simulink model "Controller_Pioneer3DXAssembly_org"  (Simulink 10.0)
settings: Solver=ode45  StartTime=0.0  StopTime=200  RelTol=1e-3  EnableMultiTasking=on
InitFcn:
  | load WorldLUTData.mat
  | r = 0.095; %Wheel radius
  | b = 0.33; %Wheel base
undefined symbols (not defined in the file): World_LUT, X, Y, Z
libraries: sm_lib x35, nesl_utility x19, fl_lib x3, fl_ps_legacy_lib x3, vrlib x2
(part 1 of 2)
settings Model: Creator=sseshadr  LastModifiedBy=bhisma
settings DataIOCC: LimitDataPoints=on
settings DebuggingCC: SolverPrmCheckMsg=warning
settings GRTTargetCC: GeneratePreprocessorConditionals=Disable all  CombineOutputUpdateFcns=on  GRTInterface=off
settings ConfigComp: CovExternalEMLEnable=off
settings SimscapeCC: SimscapeNormalizeSystem=off
settings ConfigurationSet: Description=SimMechanics 2G
settings ExplorerConfigSet: SimMechanicsOpenEditorOnUpdate=off

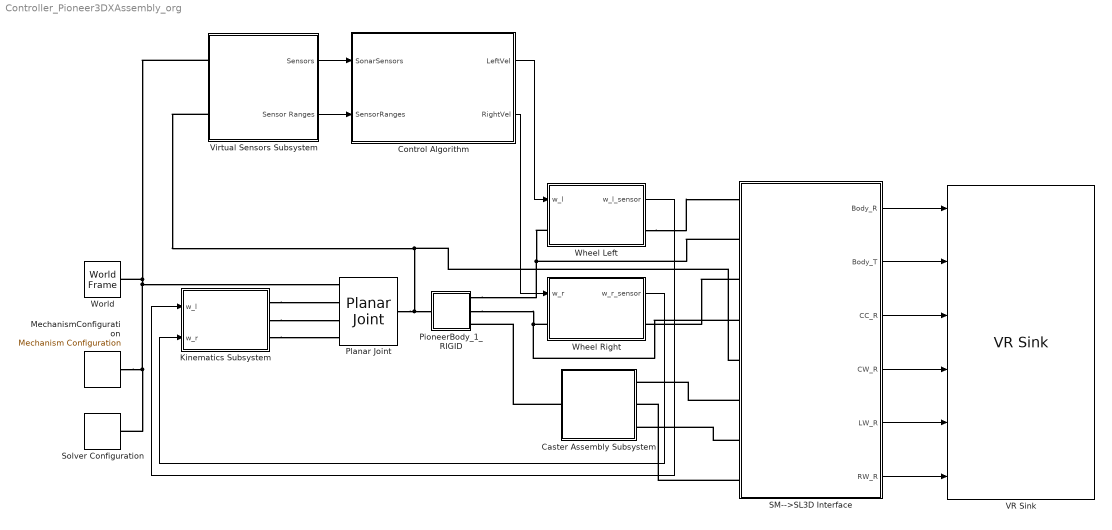
== system Controller_Pioneer3DXAssembly_org ==
  Caster Assembly Subsystem : Subsystem
  Control Algorithm : Stateflow chart  TreatAsAtomicUnit=on  mask{v0=1}
      mask prompts: v0 "Wheel Angular Velocity"
  Kinematics Subsystem : Subsystem
  MechanismConfiguration : sm_lib/Utilities/Mechanism Configuration  UniformGravity=Constant  GravityVector=[0 0 -9.81]  GravityUnits=m/s^2  LinearizationDelta=0.001
  PioneerBody_1_RIGID : Subsystem
  Planar Joint : sm_lib/Joints/Planar Joint  JointMode=Normal  SenseConstraintForce=off  SenseConstraintForceX=off  SenseConstraintForceY=off  SenseConstraintForceZ=off  SenseConstraintTorque=off  SenseConstraintTorqueX=off  SenseConstraintTorqueY=off  SenseConstraintTorqueZ=off  SenseTotalForce=off  SenseTotalForceX=off  SenseTotalForceY=off  SenseTotalForceZ=off  SenseTotalTorque=off  SenseTotalTorqueX=off  SenseTotalTorqueY=off  SenseTotalTorqueZ=off  CompositeWrenchDir=FollowerOnBase  CompositeWrenchFrame=BaseFrame  PxEquilibriumPosition=0  PxEquilibriumPositionUnits=m  PxSpringStiffness=0  PxSpringStiffnessUnits=N/m  PxDampingCoefficient=0  PxDampingCoefficientUnits=N/(m/s)  PxTorqueActuationMode=ComputedTorque  PxMotionActuationMode=InputMotion  PxSensePosition=off  PxSenseVelocity=off  PxSenseAcceleration=off  PxSenseTorqueForce=off  PxSenseLowerLimitTorqueForce=off  PxSenseUpperLimitTorqueForce=off  PxLowerLimitSpecify=off  PxLowerLimitBound=-1  PxLowerLimitBoundUnits=m  PxLowerLimitStiffness=1e6  PxLowerLimitStiffnessUnits=N/m  PxLowerLimitDamping=1e3  PxLowerLimitDampingUnits=N/(m/s)  PxLowerLimitTransitionRegionWidth=1e-4  PxLowerLimitTransitionRegionWidthUnits=m  PxUpperLimitSpecify=off  PxUpperLimitBound=1  PxUpperLimitBoundUnits=m  PxUpperLimitStiffness=1e6  PxUpperLimitStiffnessUnits=N/m  PxUpperLimitDamping=1e3  PxUpperLimitDampingUnits=N/(m/s)  PxUpperLimitTransitionRegionWidth=1e-4  PxUpperLimitTransitionRegionWidthUnits=m  PxPositionTargetSpecify=off  PxPositionTargetPriority=High  PxPositionTargetValue=0  PxPositionTargetValueUnits=m  PxVelocityTargetSpecify=off  PxVelocityTargetPriority=High  PxVelocityTargetValue=0  PxVelocityTargetValueUnits=m/s  PyEquilibriumPosition=0  PyEquilibriumPositionUnits=m  PySpringStiffness=0  PySpringStiffnessUnits=N/m  PyDampingCoefficient=0  PyDampingCoefficientUnits=N/(m/s)  PyTorqueActuationMode=ComputedTorque  PyMotionActuationMode=InputMotion  PySensePosition=off  PySenseVelocity=off  PySenseAcceleration=off  PySenseTorqueForce=off  PySenseLowerLimitTorqueForce=off  PySenseUpperLimitTorqueForce=off  PyLowerLimitSpecify=off  PyLowerLimitBound=-1  PyLowerLimitBoundUnits=m  PyLowerLimitStiffness=1e6  PyLowerLimitStiffnessUnits=N/m  PyLowerLimitDamping=1e3  PyLowerLimitDampingUnits=N/(m/s)  PyLowerLimitTransitionRegionWidth=1e-4  PyLowerLimitTransitionRegionWidthUnits=m  PyUpperLimitSpecify=off  PyUpperLimitBound=1  PyUpperLimitBoundUnits=m  PyUpperLimitStiffness=1e6  PyUpperLimitStiffnessUnits=N/m  PyUpperLimitDamping=1e3  PyUpperLimitDampingUnits=N/(m/s)  PyUpperLimitTransitionRegionWidth=1e-4  PyUpperLimitTransitionRegionWidthUnits=m  PyPositionTargetSpecify=off  PyPositionTargetPriority=High  PyPositionTargetValue=0  PyPositionTargetValueUnits=m  PyVelocityTargetSpecify=off  PyVelocityTargetPriority=High  PyVelocityTargetValue=0  PyVelocityTargetValueUnits=m/s  RzEquilibriumPosition=0  RzEquilibriumPositionUnits=deg  RzSpringStiffness=0  RzSpringStiffnessUnits=N*m/deg  RzDampingCoefficient=0  RzDampingCoefficientUnits=N*m/(deg/s)  RzTorqueActuationMode=ComputedTorque  RzMotionActuationMode=InputMotion  RzSensePosition=off  RzSenseVelocity=off  RzSenseAcceleration=off  RzSenseTorqueForce=off  RzSenseLowerLimitTorqueForce=off  RzSenseUpperLimitTorqueForce=off  RzLowerLimitSpecify=off  RzLowerLimitBound=-90  RzLowerLimitBoundUnits=deg  RzLowerLimitStiffness=1e4  RzLowerLimitStiffnessUnits=N*m/deg  RzLowerLimitDamping=10  RzLowerLimitDampingUnits=N*m/(deg/s)  RzLowerLimitTransitionRegionWidth=0.1  RzLowerLimitTransitionRegionWidthUnits=deg  RzUpperLimitSpecify=off  RzUpperLimitBound=90  RzUpperLimitBoundUnits=deg  RzUpperLimitStiffness=1e4  RzUpperLimitStiffnessUnits=N*m/deg  RzUpperLimitDamping=10  RzUpperLimitDampingUnits=N*m/(deg/s)  RzUpperLimitTransitionRegionWidth=0.1  RzUpperLimitTransitionRegionWidthUnits=deg  RzPositionTargetSpecify=off  RzPositionTargetPriority=High  RzPositionTargetValue=0  RzPositionTargetValueUnits=deg  RzVelocityTargetSpecify=off  RzVelocityTargetPriority=High  RzVelocityTargetValue=0  RzVelocityTargetValueUnits=deg/s
  SM-->SL3D Interface : Subsystem
  Solver Configuration : nesl_utility/Solver Configuration  PhysicalDomain=network_engine_domain  SubClassName=solver  LeftPortType=input  RightPortType=generic  Tones=[]  Harmonics=[]  SimulateNoise=off  Profile=off  UseLocalSampling=off  EnableSwitchedLinearOptims=on  FrequencyDomain=off  UseCCode=off  RelTol=0.001  AbsTol=1e-06  MinStep=1e-09  ToWorkspace=off  RevertToSquareIcSolve=off  NumHomotopyIterations=100  PhasorMode=off  PhasorModeNumHarmonics=1  DoDC=off  ResidualTolerance=1e-09  UseLocalSolver=off  LocalSolverChoice=NE_BACKWARD_EULER_ADVANCER  LocalSolverSampleTime=0.001  DoFixedCost=off  MaxNonlinIter=3  MaxModeIter=2  LinearAlgebra=Sparse  EquationFormulation=NE_TIME_EF  DelaysMemoryBudget=1024  AutomaticFiltering=on  FilteringTimeConstant=0.001  PartitionStorageMethod=AS_NEEDED  PartitionMemoryBudget=1024  PartitionMethod=FAST
  VR Sink : vrlib/VR Sink  InstantiateOnLoad=on  SampleTime=0.1  ViewEnable=on  RemoteChange=off  RemoteView=off  FieldsWritten=Body.rotation.4.1.1.double#Body.translation.3.1.1.double#CasterClamp.rotation.4.1.1.double#CasterWheel.rotation.4.1.1.double#LeftWheel.rotation.4.1.1.double#RightWheel.rotation.4.1.1.double  WorldFileName=PioneerWorldColor.wrl  AutoView=off  VideoDimensions=[]  AllowVariableSize=off  FigureProperties="{'Position', 'Name', 'Viewpoint', 'CameraBound', 'CameraDirection', 'CameraPosition', 'CameraUpVector', 'ZoomFactor', 'Antialiasing', 'Headlight', 'Lighting', 'NavPanel', 'StatusBar', 'ToolBar', 'Textures', 'Transparency', 'Triad', 'Wireframe', 'NavZones', 'NavMode', 'NavSpeed', 'CaptureFileFormat', 'CaptureFileName', 'Record2DCompressMethod', 'Record2DCompressQuality', 'Record2D', 'Record2DFileName', 'Record2DFPS'; [9.6500000000000000e+02   7.0000000000000000e+01   9.5200000000000000e+02   1.0310000000000000e+03], '', 'Env Front Near', 'on', [0.0000000000000000e+00   0.0000000000000000e+00  -1.0000000000000000e+00], [0.0000000000000000e+00   0.0000000000000000e+00   0.0000000000000000e+00], [0.0000000000000000e+00   1.0000000000000000e+00   0.0000000000000000e+00], [1.0000000000000000e+00], 'on', 'on', 'on', 'halfbar', 'on', 'on', 'on', 'on', 'none', 'off', 'off', 'fly', 'normal', 'tif', '%f_anim_%n.tif', 'auto', [7.5000000000000000e+01], 'off', '%f_anim_%n.avi', [1.5000000000000000e+01]}"
      settings: SourceProductName=Simulink
  Virtual Sensors Subsystem : Subsystem  mask{r_range=[450;500;500;500;500;500;500;450]}
      mask prompts: r_range "Range"
      mask DialogControl DescGroupVar Prompt: Virtual Sensors Subsystem
      mask DialogControl DescTextVar Prompt: Enter SONAR Range for the front sensors left to right as an array for in millimeters for e.g. [250;500;500;500;500;500;500;250]
  Wheel Left : Subsystem
  Wheel Right : Subsystem
  World : sm_lib/Frames and Transforms/World Frame
  wires:
  Control Algorithm/1(LeftVel) -> Wheel Left/1(w_l)
  Control Algorithm/2(RightVel) -> Wheel Right/1(w_r)
  Wheel Left/1(w_l_sensor) -> Kinematics Subsystem/1(w_l)
  Wheel Right/1(w_r_sensor) -> Kinematics Subsystem/2(w_r)
  Virtual Sensors Subsystem/1(Sensors) -> Control Algorithm/1(SonarSensors)
  Virtual Sensors Subsystem/2(Sensor Ranges) -> Control Algorithm/2(SensorRanges)
  SM-->SL3D Interface/1(Body_R) -> VR Sink/1
  SM-->SL3D Interface/6(RW_R) -> VR Sink/6
  SM-->SL3D Interface/5(LW_R) -> VR Sink/5
  SM-->SL3D Interface/3(CC_R) -> VR Sink/3
  SM-->SL3D Interface/4(CW_R) -> VR Sink/4
  SM-->SL3D Interface/2(Body_T) -> VR Sink/2
  connections:
  MechanismConfiguration/RConn1 -- Virtual Sensors Subsystem/LConn1 -- World/RConn1 -- Planar Joint/LConn1 -- Solver Configuration/RConn1
  PioneerBody_1_RIGID/RConn2 -- SM-->SL3D Interface/LConn4 -- Wheel Right/LConn1
  PioneerBody_1_RIGID/RConn1 -- Wheel Left/LConn1 -- SM-->SL3D Interface/LConn2
  Planar Joint/RConn1 -- SM-->SL3D Interface/LConn5 -- Virtual Sensors Subsystem/LConn2 -- PioneerBody_1_RIGID/LConn1
  Caster Assembly Subsystem/LConn1 -- PioneerBody_1_RIGID/RConn3
  Kinematics Subsystem/RConn1 -- Planar Joint/LConn2
  Kinematics Subsystem/RConn2 -- Planar Joint/LConn3
  Kinematics Subsystem/RConn3 -- Planar Joint/LConn4
  Wheel Left/RConn1 -- SM-->SL3D Interface/LConn1
  SM-->SL3D Interface/LConn3 -- Wheel Right/RConn1
  SM-->SL3D Interface/LConn6 -- Caster Assembly Subsystem/RConn1
  SM-->SL3D Interface/LConn8 -- Caster Assembly Subsystem/RConn2
  SM-->SL3D Interface/LConn7 -- Caster Assembly Subsystem/RConn3

== system Controller_Pioneer3DXAssembly_org/Caster Assembly Subsystem ==
  CasterWheelBody_1_RIGID : Subsystem
  CasterWheelClamp_1_RIGID : Subsystem
  Revolute : sm_lib/Joints/Revolute Joint  JointMode=Normal  SenseConstraintForce=off  SenseConstraintForceX=off  SenseConstraintForceY=off  SenseConstraintForceZ=off  SenseConstraintTorque=off  SenseConstraintTorqueX=off  SenseConstraintTorqueY=off  SenseConstraintTorqueZ=off  SenseTotalForce=off  SenseTotalForceX=off  SenseTotalForceY=off  SenseTotalForceZ=off  SenseTotalTorque=off  SenseTotalTorqueX=off  SenseTotalTorqueY=off  SenseTotalTorqueZ=off  CompositeWrenchDir=FollowerOnBase  CompositeWrenchFrame=BaseFrame  EquilibriumPosition=0  EquilibriumPositionUnits=rad  SpringStiffness=0  SpringStiffnessUnits=m*N/rad  DampingCoefficient=0  DampingCoefficientUnits=m*s*N/rad  TorqueActuationMode=NoTorque  MotionActuationMode=ComputedMotion  SensePosition=off  SenseVelocity=off  SenseAcceleration=off  SenseTorqueForce=off  SenseLowerLimitTorqueForce=off  SenseUpperLimitTorqueForce=off  LowerLimitSpecify=off  LowerLimitBound=-90  LowerLimitBoundUnits=deg  LowerLimitStiffness=1e4  LowerLimitStiffnessUnits=N*m/deg  LowerLimitDamping=10  LowerLimitDampingUnits=N*m/(deg/s)  LowerLimitTransitionRegionWidth=0.1  LowerLimitTransitionRegionWidthUnits=deg  UpperLimitSpecify=off  UpperLimitBound=90  UpperLimitBoundUnits=deg  UpperLimitStiffness=1e4  UpperLimitStiffnessUnits=N*m/deg  UpperLimitDamping=10  UpperLimitDampingUnits=N*m/(deg/s)  UpperLimitTransitionRegionWidth=0.1  UpperLimitTransitionRegionWidthUnits=deg  PositionTargetSpecify=on  PositionTargetPriority=Low  PositionTargetValue=0.2241061767810246  PositionTargetValueUnits=deg  VelocityTargetSpecify=off  VelocityTargetPriority=High  VelocityTargetValue=0  VelocityTargetValueUnits=deg/s
  Revolute1 : sm_lib/Joints/Revolute Joint  JointMode=Normal  SenseConstraintForce=off  SenseConstraintForceX=off  SenseConstraintForceY=off  SenseConstraintForceZ=off  SenseConstraintTorque=off  SenseConstraintTorqueX=off  SenseConstraintTorqueY=off  SenseConstraintTorqueZ=off  SenseTotalForce=off  SenseTotalForceX=off  SenseTotalForceY=off  SenseTotalForceZ=off  SenseTotalTorque=off  SenseTotalTorqueX=off  SenseTotalTorqueY=off  SenseTotalTorqueZ=off  CompositeWrenchDir=FollowerOnBase  CompositeWrenchFrame=BaseFrame  EquilibriumPosition=0  EquilibriumPositionUnits=rad  SpringStiffness=0  SpringStiffnessUnits=m*N/rad  DampingCoefficient=0  DampingCoefficientUnits=m*s*N/rad  TorqueActuationMode=NoTorque  MotionActuationMode=ComputedMotion  SensePosition=off  SenseVelocity=off  SenseAcceleration=off  SenseTorqueForce=off  SenseLowerLimitTorqueForce=off  SenseUpperLimitTorqueForce=off  LowerLimitSpecify=off  LowerLimitBound=-90  LowerLimitBoundUnits=deg  LowerLimitStiffness=1e4  LowerLimitStiffnessUnits=N*m/deg  LowerLimitDamping=10  LowerLimitDampingUnits=N*m/(deg/s)  LowerLimitTransitionRegionWidth=0.1  LowerLimitTransitionRegionWidthUnits=deg  UpperLimitSpecify=off  UpperLimitBound=90  UpperLimitBoundUnits=deg  UpperLimitStiffness=1e4  UpperLimitStiffnessUnits=N*m/deg  UpperLimitDamping=10  UpperLimitDampingUnits=N*m/(deg/s)  UpperLimitTransitionRegionWidth=0.1  UpperLimitTransitionRegionWidthUnits=deg  PositionTargetSpecify=on  PositionTargetPriority=Low  PositionTargetValue=0.06600758954149441  PositionTargetValueUnits=deg  VelocityTargetSpecify=off  VelocityTargetPriority=High  VelocityTargetValue=0  VelocityTargetValueUnits=deg/s
  CWCA : PMIOPort  Side=Left
  CWC : PMIOPort  Port=2  Side=Right
  CWBA : PMIOPort  Port=3  Side=Right
  CWB : PMIOPort  Port=4  Side=Right
  connections:
  Revolute1/LConn1 -- CWBA/RConn1 -- CasterWheelClamp_1_RIGID/RConn1
  CWCA/RConn1 -- Revolute/LConn1
  Revolute1/RConn1 -- CWB/RConn1 -- CasterWheelBody_1_RIGID/LConn1
  Revolute/RConn1 -- CWC/RConn1 -- CasterWheelClamp_1_RIGID/LConn1

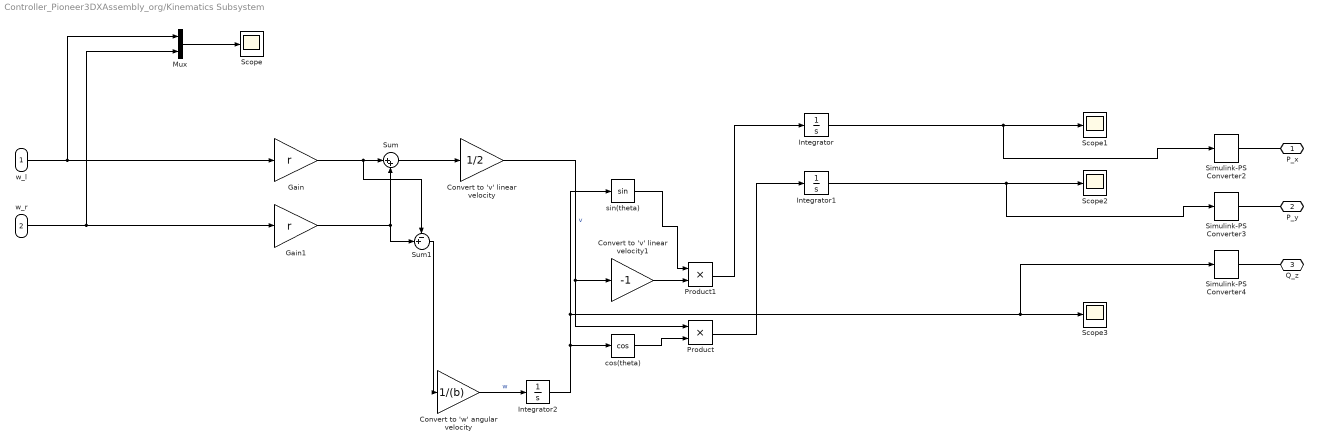
== system Controller_Pioneer3DXAssembly_org/Kinematics Subsystem ==
  w_l : Inport
  w_r : Inport  Port=2
  Convert to 'v' linear velocity : Gain  Gain=1/2
  Convert to 'v' linear velocity1 : Gain  Gain=-1
  Convert to 'w' angular velocity : Gain  Gain=1/(b)
  Gain : Gain  Gain=r
  Gain1 : Gain  Gain=r
  Integrator : Integrator
  Integrator1 : Integrator
  Integrator2 : Integrator
  Mux : Mux  Inputs=2
  Product : Product
  Product1 : Product
  Scope{,1..3} (4 alike) : Scope
  Simulink-PS Converter2 : nesl_utility/Simulink-PS Converter  PhysicalDomain=network_engine_domain  SubClassName=ps_input  LeftPortType=input  RightPortType=output  PseudoPeriodic=off  Frequencies=[]  NoiseDistribution=none  NoiseParameters=[]  Unit=1  AffineConversion=off  FilteringAndDerivatives=filter  SimscapeFilterOrder=2  InputFilterTimeConstant=0.01  UdotUserProvided=1
  Simulink-PS Converter3 : nesl_utility/Simulink-PS Converter  PhysicalDomain=network_engine_domain  SubClassName=ps_input  LeftPortType=input  RightPortType=output  PseudoPeriodic=off  Frequencies=[]  NoiseDistribution=none  NoiseParameters=[]  Unit=1  AffineConversion=off  FilteringAndDerivatives=filter  SimscapeFilterOrder=2  InputFilterTimeConstant=0.01  UdotUserProvided=1
  Simulink-PS Converter4 : nesl_utility/Simulink-PS Converter  PhysicalDomain=network_engine_domain  SubClassName=ps_input  LeftPortType=input  RightPortType=output  PseudoPeriodic=off  Frequencies=[]  NoiseDistribution=none  NoiseParameters=[]  Unit=1  AffineConversion=off  FilteringAndDerivatives=filter  SimscapeFilterOrder=2  InputFilterTimeConstant=0.01  UdotUserProvided=1
  Sum : Sum  Inputs=|++
  Sum1 : Sum  Inputs=-+|
  cos(theta) : Trigonometry  Operator=cos
  sin(theta) : Trigonometry
  P_x : PMIOPort  Side=Right
  P_y : PMIOPort  Port=2  Side=Right
  Q_z : PMIOPort  Port=3  Side=Right
  wires:
  Convert to 'v' linear velocity1/1 -> Product1/2
  Mux/1 -> Scope/1
  Product/1 -> Integrator1/1
  Product1/1 -> Integrator/1
  w_r/1 -> Gain1/1, Mux/2
  w_l/1 -> Gain/1, Mux/1
  Convert to 'v' linear velocity/1 -> Product/1, Convert to 'v' linear velocity1/1  "v"
  Sum1/1 -> Convert to 'w' angular velocity/1
  cos(theta)/1 -> Product/2
  sin(theta)/1 -> Product1/1
  Integrator2/1 -> cos(theta)/1, sin(theta)/1, Scope3/1, Simulink-PS Converter4/1
  Convert to 'w' angular velocity/1 -> Integrator2/1  "w"
  Integrator1/1 -> Scope2/1, Simulink-PS Converter3/1
  Integrator/1 -> Scope1/1, Simulink-PS Converter2/1
  Sum/1 -> Convert to 'v' linear velocity/1
  Gain/1 -> Sum/1, Sum1/1
  Gain1/1 -> Sum1/2, Sum/2
  connections:
  Simulink-PS Converter3/RConn1 -- P_y/RConn1
  Simulink-PS Converter2/RConn1 -- P_x/RConn1
  Simulink-PS Converter4/RConn1 -- Q_z/RConn1

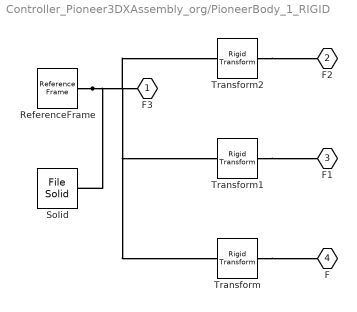
== system Controller_Pioneer3DXAssembly_org/PioneerBody_1_RIGID ==
  ReferenceFrame : sm_lib/Frames and Transforms/Reference Frame
  Solid : sm_lib/Body Elements/File Solid  ExtGeomFileName=PioneerBody_Default_sldprt.STL  UnitType=FromFile  ExtGeomFileUnits=in  StepReaderType=HEX  ExportEntireGeometry=off  InertiaType=Custom  Mass=6.1597799999999996  MassUnits=kg  CenterOfMass=[0.18851259842519683 -1.4327086614173226 1.4471535433070863]  CenterOfMassUnits=in  MomentsOfInertia=[221.24124248248489 141.00548701097398 265.04278008556008]  MomentsOfInertiaUnits=kg*in^2  ProductsOfInertia=[-5.571098642197283 -0.58057691115382204 1.1589822679645356]  ProductsOfInertiaUnits=kg*in^2  BasedOnType=Density  Density=1000  DensityUnits=kg/(m^3)  DoExposeReferenceFrame=on  SerializedFrames=<Frames/>  GraphicType=FromGeometry  MarkerShape=Sphere  MarkerSize=10  MarkerSizeUnits=m  GraphicVisPropType=SimpleVisualProperties  GraphicDiffuseColor=[0.866667 0.909804 1]  GraphicSpecularColor=[0.5 0.5 0.5 1.0]  GraphicAmbientColor=[0.15 0.15 0.15 1.0]  GraphicEmissiveColor=[0.0 0.0 0.0 1.0]  GraphicShininess=75  GraphicOpacity=1
  Transform : sm_lib/Frames and Transforms/Rigid Transform  TranslationMethod=Cartesian  TranslationStandardOffset=0  TranslationLengthUnit=m  TranslationStandardAxis=+Z  TranslationCartesianOffset=[0.0050419000000000002 -0.181229 -0.0009905999999999999]  TranslationROffset=0  TranslationROffsetUnits=m  TranslationZOffset=0  TranslationZOffsetUnits=m  TranslationThetaOffset=0  TranslationThetaOffsetUnits=deg  RotationMethod=ArbitraryAxis  RotationAngleUnits=rad  RotationStandardAxis=+Z  RotationAngle=0  RotationArbitraryAxis=[0 0 0]  FollAlignAxisA=+X  BaseAlignAxisA=+Y  FollAlignAxisB=+Y  BaseAlignAxisB=+Z  RotationSequenceAxes=FollowerAxes  RotationSequence=XYX  RotationSequenceAngles=[0 0 0]  RotationSequenceAnglesUnits=deg  RotationMatrix=[1 0 0; 0 1 0; 0 0 1]
  Transform1 : sm_lib/Frames and Transforms/Rigid Transform  TranslationMethod=Cartesian  TranslationStandardOffset=0  TranslationLengthUnit=m  TranslationStandardAxis=+Z  TranslationCartesianOffset=[0.189166 2.4979999999999999e-16 0.0016256]  TranslationROffset=0  TranslationROffsetUnits=m  TranslationZOffset=0  TranslationZOffsetUnits=m  TranslationThetaOffset=0  TranslationThetaOffsetUnits=deg  RotationMethod=ArbitraryAxis  RotationAngleUnits=rad  RotationStandardAxis=+Z  RotationAngle=2.0943951023931957  RotationArbitraryAxis=[-0.57735026918962573 -0.57735026918962584 0.57735026918962573]  FollAlignAxisA=+X  BaseAlignAxisA=+Y  FollAlignAxisB=+Y  BaseAlignAxisB=+Z  RotationSequenceAxes=FollowerAxes  RotationSequence=XYX  RotationSequenceAngles=[0 0 0]  RotationSequenceAnglesUnits=deg  RotationMatrix=[1 0 0; 0 1 0; 0 0 1]
  Transform2 : sm_lib/Frames and Transforms/Rigid Transform  TranslationMethod=Cartesian  TranslationStandardOffset=0  TranslationLengthUnit=m  TranslationStandardAxis=+Z  TranslationCartesianOffset=[-0.17908299999999999 0 0.0016256]  TranslationROffset=0  TranslationROffsetUnits=m  TranslationZOffset=0  TranslationZOffsetUnits=m  TranslationThetaOffset=0  TranslationThetaOffsetUnits=deg  RotationMethod=ArbitraryAxis  RotationAngleUnits=rad  RotationStandardAxis=+Z  RotationAngle=2.0943951023931953  RotationArbitraryAxis=[0.57735026918962562 0.57735026918962562 0.57735026918962595]  FollAlignAxisA=+X  BaseAlignAxisA=+Y  FollAlignAxisB=+Y  BaseAlignAxisB=+Z  RotationSequenceAxes=FollowerAxes  RotationSequence=XYX  RotationSequenceAngles=[0 0 0]  RotationSequenceAnglesUnits=deg  RotationMatrix=[1 0 0; 0 1 0; 0 0 1]
  F3 : PMIOPort  Side=Left
  F2 : PMIOPort  Port=2  Side=Right
  F1 : PMIOPort  Port=3  Side=Right
  F : PMIOPort  Port=4  Side=Right
  connections:
  Solid/RConn1 -- ReferenceFrame/RConn1 -- Transform/LConn1 -- Transform1/LConn1 -- Transform2/LConn1 -- F3/RConn1
  Transform/RConn1 -- F/RConn1
  Transform1/RConn1 -- F1/RConn1
  Transform2/RConn1 -- F2/RConn1

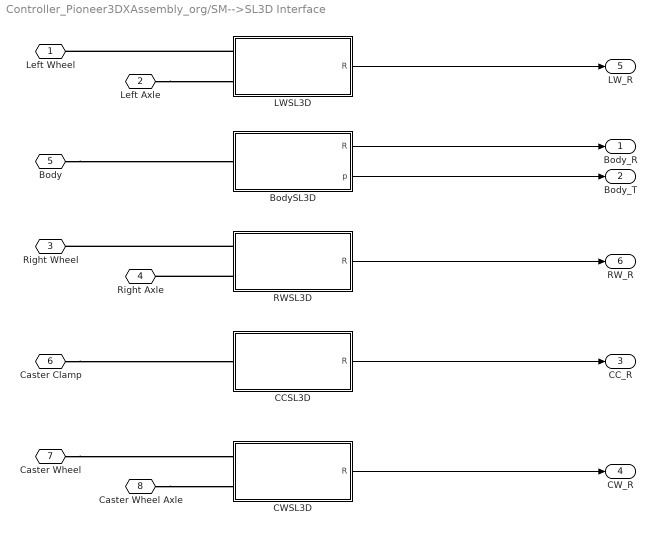
== system Controller_Pioneer3DXAssembly_org/SM-->SL3D Interface ==
  "BodySL3D " : Subsystem
  CCSL3D : Subsystem
  CWSL3D : Subsystem
  LWSL3D : Subsystem
  RWSL3D : Subsystem
  Left Wheel : PMIOPort  Side=Left
  Left Axle : PMIOPort  Port=2  Side=Left
  Right Wheel : PMIOPort  Port=3  Side=Left
  Right Axle : PMIOPort  Port=4  Side=Left
  Body : PMIOPort  Port=5  Side=Left
  Caster Clamp : PMIOPort  Port=6  Side=Left
  Caster Wheel : PMIOPort  Port=7  Side=Left
  Caster Wheel Axle : PMIOPort  Port=8  Side=Left
  Body_R : Outport
  Body_T : Outport  Port=2
  CC_R : Outport  Port=3
  CW_R : Outport  Port=4
  LW_R : Outport  Port=5
  RW_R : Outport  Port=6
  wires:
  "BodySL3D "/1(R) -> Body_R/1
  "BodySL3D "/2(p) -> Body_T/1
  CWSL3D/1(R) -> CW_R/1
  CCSL3D/1(R) -> CC_R/1
  RWSL3D/1(R) -> RW_R/1
  LWSL3D/1(R) -> LW_R/1
  connections:
  Caster Wheel Axle/RConn1 -- CWSL3D/LConn2
  RWSL3D/LConn2 -- Right Axle/RConn1
  Left Axle/RConn1 -- LWSL3D/LConn2
  Body/RConn1 -- "BodySL3D "/LConn1
  Caster Clamp/RConn1 -- CCSL3D/LConn1
  Caster Wheel/RConn1 -- CWSL3D/LConn1
  RWSL3D/LConn1 -- Right Wheel/RConn1
  LWSL3D/LConn1 -- Left Wheel/RConn1

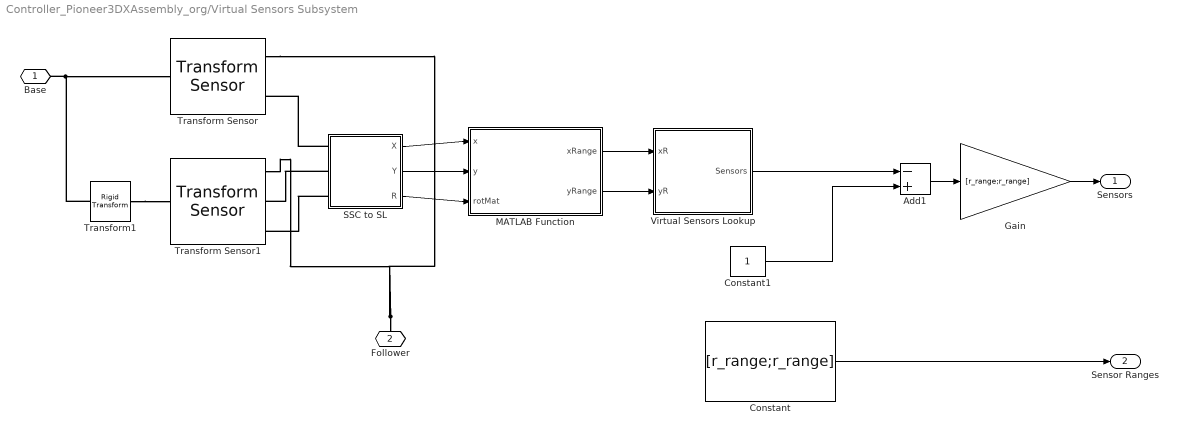
== system Controller_Pioneer3DXAssembly_org/Virtual Sensors Subsystem ==
  Add1 : Sum  Inputs=-+
  Constant : Constant  Value=[r_range;r_range]
  Constant1 : Constant
  Gain : Gain  Gain=[r_range;r_range]
  MATLAB Function : MATLAB Function  TreatAsAtomicUnit=on
  SSC to SL : Subsystem
  Transform Sensor : sm_lib/Frames and Transforms/Transform Sensor  MeasurementFrame=Base  SenseAngle=off  SenseAxis=off  SenseAngle1=off  SenseAngle2=off  SenseAngle3=off  SenseQ=off  SenseR=on  SenseOmegaX=off  SenseOmegaY=off  SenseOmegaZ=off  SenseOmega1=off  SenseOmega2=off  SenseOmega3=off  SenseQDot=off  SenseRDot=off  SenseAlphaX=off  SenseAlphaY=off  SenseAlphaZ=off  SenseAlpha1=off  SenseAlpha2=off  SenseAlpha3=off  SenseQDDot=off  SenseRDDot=off  SenseX=off  SenseY=off  SenseZ=off  SenseRad=off  SenseAzim=off  SenseDist=off  SenseInc=off  SenseXDot=off  SenseYDot=off  SenseZDot=off  SenseRadDot=off  SenseAzimDot=off  SenseDistDot=off  SenseIncDot=off  SenseXDDot=off  SenseYDDot=off  SenseZDDot=off  SenseRadDDot=off  SenseAzimDDot=off  SenseDistDDot=off  SenseIncDDot=off
  Transform Sensor1 : sm_lib/Frames and Transforms/Transform Sensor  MeasurementFrame=Base  SenseAngle=off  SenseAxis=off  SenseAngle1=off  SenseAngle2=off  SenseAngle3=off  SenseQ=off  SenseR=off  SenseOmegaX=off  SenseOmegaY=off  SenseOmegaZ=off  SenseOmega1=off  SenseOmega2=off  SenseOmega3=off  SenseQDot=off  SenseRDot=off  SenseAlphaX=off  SenseAlphaY=off  SenseAlphaZ=off  SenseAlpha1=off  SenseAlpha2=off  SenseAlpha3=off  SenseQDDot=off  SenseRDDot=off  SenseX=on  SenseY=on  SenseZ=off  SenseRad=off  SenseAzim=off  SenseDist=off  SenseInc=off  SenseXDot=off  SenseYDot=off  SenseZDot=off  SenseRadDot=off  SenseAzimDot=off  SenseDistDot=off  SenseIncDot=off  SenseXDDot=off  SenseYDDot=off  SenseZDDot=off  SenseRadDDot=off  SenseAzimDDot=off  SenseDistDDot=off  SenseIncDDot=off
  Transform1 : sm_lib/Frames and Transforms/Rigid Transform  TranslationMethod=Cartesian  TranslationStandardOffset=0  TranslationLengthUnit=m  TranslationStandardAxis=+Z  TranslationCartesianOffset=[0 0 0]  TranslationROffset=0  TranslationROffsetUnits=m  TranslationZOffset=0  TranslationZOffsetUnits=m  TranslationThetaOffset=0  TranslationThetaOffsetUnits=deg  RotationMethod=StandardAxis  RotationAngleUnits=deg  RotationStandardAxis=+Z  RotationAngle=-90  RotationArbitraryAxis=[0 0 1]  FollAlignAxisA=+X  BaseAlignAxisA=+Y  FollAlignAxisB=+Y  BaseAlignAxisB=+Z  RotationSequenceAxes=FollowerAxes  RotationSequence=XYX  RotationSequenceAngles=[0 0 0]  RotationSequenceAnglesUnits=deg  RotationMatrix=[1 0 0; 0 1 0; 0 0 1]
  Virtual Sensors Lookup : Subsystem
  Base : PMIOPort  Side=Left
  Follower : PMIOPort  Port=2  Side=Left
  Sensors : Outport
  Sensor Ranges : Outport  Port=2
  wires:
  MATLAB Function/2(yRange) -> Virtual Sensors Lookup/2(yR)
  MATLAB Function/1(xRange) -> Virtual Sensors Lookup/1(xR)
  SSC to SL/3(R) -> MATLAB Function/3(rotMat)
  SSC to SL/2(Y) -> MATLAB Function/2(y)
  SSC to SL/1(X) -> MATLAB Function/1(x)
  Add1/1 -> Gain/1
  Constant/1 -> Sensor Ranges/1
  Constant1/1 -> Add1/2
  Virtual Sensors Lookup/1(Sensors) -> Add1/1
  Gain/1 -> Sensors/1
  connections:
  Transform1/RConn1 -- Transform Sensor1/LConn1
  SSC to SL/LConn2 -- Transform Sensor1/RConn2
  SSC to SL/LConn3 -- Transform Sensor1/RConn3
  SSC to SL/LConn1 -- Transform Sensor/RConn2
  Base/RConn1 -- Transform1/LConn1 -- Transform Sensor/LConn1
  Follower/RConn1 -- Transform Sensor1/RConn1 -- Transform Sensor/RConn1

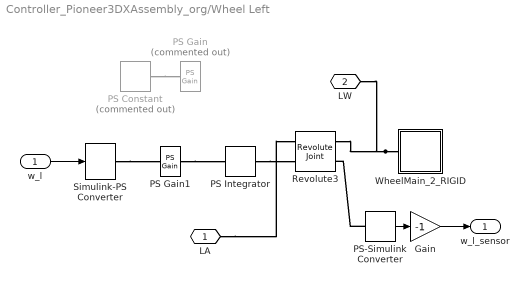
== system Controller_Pioneer3DXAssembly_org/Wheel Left ==
  w_l : Inport
  Gain : Gain  Gain=-1
  PS Constant : fl_lib/Physical Signals/Sources/PS Constant  Commented=on  constant=-0.1  LocalVarLogging=[]
  PS Gain : fl_lib/Physical Signals/Functions/PS Gain  Commented=on  gain=-1  LocalVarLogging=[]
  PS Gain1 : fl_ps_legacy_lib/Legacy Physical Signals/Functions/PS Gain  gain=-1
      settings: SourceProductName=Simscape
  PS Integrator : fl_ps_legacy_lib/Legacy Physical Signals/Linear Operators/PS Integrator  x0=0
      settings: SourceProductName=Simscape  SourceProductBaseCode=SS  InternalSimscapePortConfiguration="{\"Bottom\":[],\"Left\":[{\"id\":\"I\",\"label\":\"\",\"type\":\"input\"}],\"Right\":[{\"id\":\"O\",\"label\":\"\",\"type\":\"output\"}],\"Top\":[]}"
  PS-Simulink Converter : nesl_utility/PS-Simulink Converter  PhysicalDomain=network_engine_domain  SubClassName=ps_output  LeftPortType=input  RightPortType=output  PseudoPeriodic=off  Frequencies=[]  Unit=1  AffineConversion=off
  Revolute3 : sm_lib/Joints/Revolute Joint  JointMode=Normal  SenseConstraintForce=off  SenseConstraintForceX=off  SenseConstraintForceY=off  SenseConstraintForceZ=off  SenseConstraintTorque=off  SenseConstraintTorqueX=off  SenseConstraintTorqueY=off  SenseConstraintTorqueZ=off  SenseTotalForce=off  SenseTotalForceX=off  SenseTotalForceY=off  SenseTotalForceZ=off  SenseTotalTorque=off  SenseTotalTorqueX=off  SenseTotalTorqueY=off  SenseTotalTorqueZ=off  CompositeWrenchDir=FollowerOnBase  CompositeWrenchFrame=BaseFrame  EquilibriumPosition=0  EquilibriumPositionUnits=rad  SpringStiffness=0  SpringStiffnessUnits=m*N/rad  DampingCoefficient=0  DampingCoefficientUnits=m*s*N/rad  TorqueActuationMode=ComputedTorque  MotionActuationMode=InputMotion  SensePosition=off  SenseVelocity=on  SenseAcceleration=off  SenseTorqueForce=off  SenseLowerLimitTorqueForce=off  SenseUpperLimitTorqueForce=off  LowerLimitSpecify=off  LowerLimitBound=-90  LowerLimitBoundUnits=deg  LowerLimitStiffness=1e4  LowerLimitStiffnessUnits=N*m/deg  LowerLimitDamping=10  LowerLimitDampingUnits=N*m/(deg/s)  LowerLimitTransitionRegionWidth=0.1  LowerLimitTransitionRegionWidthUnits=deg  UpperLimitSpecify=off  UpperLimitBound=90  UpperLimitBoundUnits=deg  UpperLimitStiffness=1e4  UpperLimitStiffnessUnits=N*m/deg  UpperLimitDamping=10  UpperLimitDampingUnits=N*m/(deg/s)  UpperLimitTransitionRegionWidth=0.1  UpperLimitTransitionRegionWidthUnits=deg  PositionTargetSpecify=on  PositionTargetPriority=Low  PositionTargetValue=79.291409576446028  PositionTargetValueUnits=deg  VelocityTargetSpecify=off  VelocityTargetPriority=High  VelocityTargetValue=0  VelocityTargetValueUnits=deg/s
  Simulink-PS Converter : nesl_utility/Simulink-PS Converter  PhysicalDomain=network_engine_domain  SubClassName=ps_input  LeftPortType=input  RightPortType=output  PseudoPeriodic=off  Frequencies=[]  NoiseDistribution=none  NoiseParameters=[]  Unit=1  AffineConversion=off  FilteringAndDerivatives=zero  SimscapeFilterOrder=1  InputFilterTimeConstant=0.001  UdotUserProvided=1
  WheelMain_2_RIGID : Subsystem
  LA : PMIOPort  Side=Left
  LW : PMIOPort  Port=2  Side=Right
  w_l_sensor : Outport
  wires:
  w_l/1 -> Simulink-PS Converter/1
  Gain/1 -> w_l_sensor/1
  PS-Simulink Converter/1 -> Gain/1
  connections:
  PS Gain1/RConn1 -- PS Integrator/LConn1
  Simulink-PS Converter/RConn1 -- PS Gain1/LConn1
  PS-Simulink Converter/LConn1 -- Revolute3/RConn2
  PS Constant/RConn1 -- PS Gain/LConn1
  PS Integrator/RConn1 -- Revolute3/LConn2
  LA/RConn1 -- Revolute3/LConn1
  WheelMain_2_RIGID/LConn1 -- LW/RConn1 -- Revolute3/RConn1

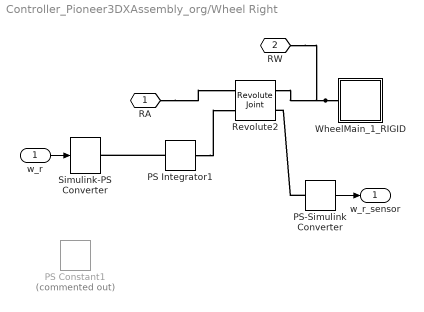
== system Controller_Pioneer3DXAssembly_org/Wheel Right ==
  w_r : Inport
  PS Constant1 : fl_lib/Physical Signals/Sources/PS Constant  Commented=on  constant=-0.1  LocalVarLogging=[]
  PS Integrator1 : fl_ps_legacy_lib/Legacy Physical Signals/Linear Operators/PS Integrator  x0=0
      settings: SourceProductName=Simscape  SourceProductBaseCode=SS  InternalSimscapePortConfiguration="{\"Bottom\":[],\"Left\":[{\"id\":\"I\",\"label\":\"\",\"type\":\"input\"}],\"Right\":[{\"id\":\"O\",\"label\":\"\",\"type\":\"output\"}],\"Top\":[]}"
  PS-Simulink Converter : nesl_utility/PS-Simulink Converter  PhysicalDomain=network_engine_domain  SubClassName=ps_output  LeftPortType=input  RightPortType=output  PseudoPeriodic=off  Frequencies=[]  Unit=1  AffineConversion=off
  Revolute2 : sm_lib/Joints/Revolute Joint  JointMode=Normal  SenseConstraintForce=off  SenseConstraintForceX=off  SenseConstraintForceY=off  SenseConstraintForceZ=off  SenseConstraintTorque=off  SenseConstraintTorqueX=off  SenseConstraintTorqueY=off  SenseConstraintTorqueZ=off  SenseTotalForce=off  SenseTotalForceX=off  SenseTotalForceY=off  SenseTotalForceZ=off  SenseTotalTorque=off  SenseTotalTorqueX=off  SenseTotalTorqueY=off  SenseTotalTorqueZ=off  CompositeWrenchDir=FollowerOnBase  CompositeWrenchFrame=BaseFrame  EquilibriumPosition=0  EquilibriumPositionUnits=rad  SpringStiffness=0  SpringStiffnessUnits=m*N/rad  DampingCoefficient=0  DampingCoefficientUnits=m*s*N/rad  TorqueActuationMode=ComputedTorque  MotionActuationMode=InputMotion  SensePosition=off  SenseVelocity=on  SenseAcceleration=off  SenseTorqueForce=off  SenseLowerLimitTorqueForce=off  SenseUpperLimitTorqueForce=off  LowerLimitSpecify=off  LowerLimitBound=-90  LowerLimitBoundUnits=deg  LowerLimitStiffness=1e4  LowerLimitStiffnessUnits=N*m/deg  LowerLimitDamping=10  LowerLimitDampingUnits=N*m/(deg/s)  LowerLimitTransitionRegionWidth=0.1  LowerLimitTransitionRegionWidthUnits=deg  UpperLimitSpecify=off  UpperLimitBound=90  UpperLimitBoundUnits=deg  UpperLimitStiffness=1e4  UpperLimitStiffnessUnits=N*m/deg  UpperLimitDamping=10  UpperLimitDampingUnits=N*m/(deg/s)  UpperLimitTransitionRegionWidth=0.1  UpperLimitTransitionRegionWidthUnits=deg  PositionTargetSpecify=on  PositionTargetPriority=Low  PositionTargetValue=37.392721804214197  PositionTargetValueUnits=deg  VelocityTargetSpecify=off  VelocityTargetPriority=High  VelocityTargetValue=0  VelocityTargetValueUnits=deg/s
  Simulink-PS Converter : nesl_utility/Simulink-PS Converter  PhysicalDomain=network_engine_domain  SubClassName=ps_input  LeftPortType=input  RightPortType=output  PseudoPeriodic=off  Frequencies=[]  NoiseDistribution=none  NoiseParameters=[]  Unit=1  AffineConversion=off  FilteringAndDerivatives=zero  SimscapeFilterOrder=1  InputFilterTimeConstant=0.001  UdotUserProvided=1
  WheelMain_1_RIGID : Subsystem
  RA : PMIOPort  Side=Left
  RW : PMIOPort  Port=2  Side=Right
  w_r_sensor : Outport
  wires:
  w_r/1 -> Simulink-PS Converter/1
  PS-Simulink Converter/1 -> w_r_sensor/1
  connections:
  PS-Simulink Converter/LConn1 -- Revolute2/RConn2
  PS Integrator1/LConn1 -- Simulink-PS Converter/RConn1
  PS Integrator1/RConn1 -- Revolute2/LConn2
  WheelMain_1_RIGID/LConn1 -- RW/RConn1 -- Revolute2/RConn1
  RA/RConn1 -- Revolute2/LConn1

== system Controller_Pioneer3DXAssembly_org/Caster Assembly Subsystem/CasterWheelBody_1_RIGID ==
  ReferenceFrame : sm_lib/Frames and Transforms/Reference Frame
  Solid : sm_lib/Body Elements/File Solid  ExtGeomFileName=CasterWheelBody_Default_sldprt.STL  UnitType=FromFile  ExtGeomFileUnits=in  StepReaderType=HEX  ExportEntireGeometry=off  InertiaType=Custom  Mass=0.165487  MassUnits=kg  CenterOfMass=[0.19849999999999998 -8.254999999999999 -2.0389999999999997]  CenterOfMassUnits=in  MomentsOfInertia=[0.17489149978299948 0.10937255874511745 0.10937255874511745]  MomentsOfInertiaUnits=kg*in^2  ProductsOfInertia=[0 0 0]  ProductsOfInertiaUnits=kg*in^2  BasedOnType=Density  Density=1000  DensityUnits=kg/(m^3)  DoExposeReferenceFrame=on  SerializedFrames=<Frames/>  GraphicType=FromGeometry  MarkerShape=Sphere  MarkerSize=10  MarkerSizeUnits=m  GraphicVisPropType=SimpleVisualProperties  GraphicDiffuseColor=[1 1 1]  GraphicSpecularColor=[0.5 0.5 0.5 1.0]  GraphicAmbientColor=[0.15 0.15 0.15 1.0]  GraphicEmissiveColor=[0.0 0.0 0.0 1.0]  GraphicShininess=75  GraphicOpacity=0.3
  Transform : sm_lib/Frames and Transforms/Rigid Transform  TranslationMethod=Cartesian  TranslationStandardOffset=0  TranslationLengthUnit=m  TranslationStandardAxis=+Z  TranslationCartesianOffset=[0.028917897723264436 -0.20967707414385042 -0.051790592740231157]  TranslationROffset=0  TranslationROffsetUnits=m  TranslationZOffset=0  TranslationZOffsetUnits=m  TranslationThetaOffset=0  TranslationThetaOffsetUnits=deg  RotationMethod=ArbitraryAxis  RotationAngleUnits=rad  RotationStandardAxis=+Z  RotationAngle=2.0943951047149336  RotationArbitraryAxis=[-0.57735026764134723 -0.57735026996353855 0.57735026996399152]  FollAlignAxisA=+X  BaseAlignAxisA=+Y  FollAlignAxisB=+Y  BaseAlignAxisB=+Z  RotationSequenceAxes=FollowerAxes  RotationSequence=XYX  RotationSequenceAngles=[0 0 0]  RotationSequenceAnglesUnits=deg  RotationMatrix=[1 0 0; 0 1 0; 0 0 1]
  F : PMIOPort  Side=Left
  connections:
  Transform/RConn1 -- F/RConn1
  Transform/LConn1 -- ReferenceFrame/RConn1 -- Solid/RConn1

== system Controller_Pioneer3DXAssembly_org/Caster Assembly Subsystem/CasterWheelClamp_1_RIGID ==
  ReferenceFrame : sm_lib/Frames and Transforms/Reference Frame
  Solid : sm_lib/Body Elements/File Solid  ExtGeomFileName=CasterWheelClamp_Default_sldprt.STL  UnitType=FromFile  ExtGeomFileUnits=in  StepReaderType=HEX  ExportEntireGeometry=off  InertiaType=Custom  Mass=0.058131799999999997  MassUnits=kg  CenterOfMass=[0.19850078740157479 -7.4364566929133851 -0.68144881889763764]  CenterOfMassUnits=in  MomentsOfInertia=[0.051037727075454134 0.062244869489738952 0.061463822927645829]  MomentsOfInertiaUnits=kg*in^2  ProductsOfInertia=[0.01403912207824415 8.7254944509888994e-09 1.0837358174716347e-07]  ProductsOfInertiaUnits=kg*in^2  BasedOnType=Density  Density=1000  DensityUnits=kg/(m^3)  DoExposeReferenceFrame=on  SerializedFrames=<Frames/>  GraphicType=FromGeometry  MarkerShape=Sphere  MarkerSize=10  MarkerSizeUnits=m  GraphicVisPropType=SimpleVisualProperties  GraphicDiffuseColor=[0.866667 0.909804 1]  GraphicSpecularColor=[0.5 0.5 0.5 1.0]  GraphicAmbientColor=[0.15 0.15 0.15 1.0]  GraphicEmissiveColor=[0.0 0.0 0.0 1.0]  GraphicShininess=75  GraphicOpacity=1
  Transform : sm_lib/Frames and Transforms/Rigid Transform  TranslationMethod=Cartesian  TranslationStandardOffset=0  TranslationLengthUnit=m  TranslationStandardAxis=+Z  TranslationCartesianOffset=[0.0050418929299438885 -0.18122900707005232 -0.00099059999999999426]  TranslationROffset=0  TranslationROffsetUnits=m  TranslationZOffset=0  TranslationZOffsetUnits=m  TranslationThetaOffset=0  TranslationThetaOffsetUnits=deg  RotationMethod=ArbitraryAxis  RotationAngleUnits=rad  RotationStandardAxis=+Z  RotationAngle=0  RotationArbitraryAxis=[0 0 0]  FollAlignAxisA=+X  BaseAlignAxisA=+Y  FollAlignAxisB=+Y  BaseAlignAxisB=+Z  RotationSequenceAxes=FollowerAxes  RotationSequence=XYX  RotationSequenceAngles=[0 0 0]  RotationSequenceAnglesUnits=deg  RotationMatrix=[1 0 0; 0 1 0; 0 0 1]
  Transform1 : sm_lib/Frames and Transforms/Rigid Transform  TranslationMethod=Cartesian  TranslationStandardOffset=0  TranslationLengthUnit=m  TranslationStandardAxis=+Z  TranslationCartesianOffset=[0.0289179 -0.209677 -0.051790599999999999]  TranslationROffset=0  TranslationROffsetUnits=m  TranslationZOffset=0  TranslationZOffsetUnits=m  TranslationThetaOffset=0  TranslationThetaOffsetUnits=deg  RotationMethod=ArbitraryAxis  RotationAngleUnits=rad  RotationStandardAxis=+Z  RotationAngle=2.0943951023931957  RotationArbitraryAxis=[-0.57735026918962573 -0.57735026918962584 0.57735026918962573]  FollAlignAxisA=+X  BaseAlignAxisA=+Y  FollAlignAxisB=+Y  BaseAlignAxisB=+Z  RotationSequenceAxes=FollowerAxes  RotationSequence=XYX  RotationSequenceAngles=[0 0 0]  RotationSequenceAnglesUnits=deg  RotationMatrix=[1 0 0; 0 1 0; 0 0 1]
  F : PMIOPort  Side=Left
  F1 : PMIOPort  Port=2  Side=Right
  connections:
  Transform1/RConn1 -- F1/RConn1
  Transform/RConn1 -- F/RConn1
  Transform1/LConn1 -- Transform/LConn1 -- ReferenceFrame/RConn1 -- Solid/RConn1

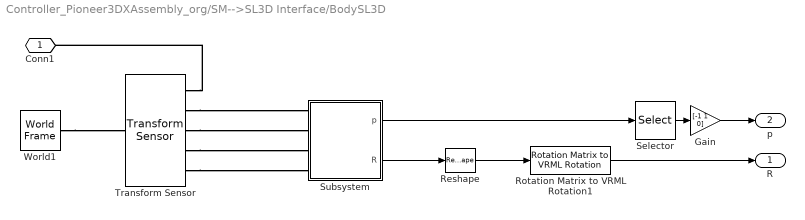
== system Controller_Pioneer3DXAssembly_org/SM-->SL3D Interface/BodySL3D  ==
  Gain : Gain  Gain=[-1 1 0]
  Reshape : Reshape  OutputDimensionality=Customize  OutputDimensions=[3 3]
  Rotation Matrix to VRML Rotation1 : vrlib/Utilities/Rotation Matrix to VRML Rotation  maxzero=1e-12
      settings: SourceProductName=Simulink  SourceProductBaseCode=SL
  Selector : Selector  InputPortWidth=3  IndexOptions=Index vector (dialog)  Indices=[2 1 3]  OutputSizes=1
  Subsystem : Subsystem
  Transform Sensor : sm_lib/Frames and Transforms/Transform Sensor  MeasurementFrame=World  SenseAngle=off  SenseAxis=off  SenseAngle1=off  SenseAngle2=off  SenseAngle3=off  SenseQ=off  SenseR=on  SenseOmegaX=off  SenseOmegaY=off  SenseOmegaZ=off  SenseOmega1=off  SenseOmega2=off  SenseOmega3=off  SenseQDot=off  SenseRDot=off  SenseAlphaX=off  SenseAlphaY=off  SenseAlphaZ=off  SenseAlpha1=off  SenseAlpha2=off  SenseAlpha3=off  SenseQDDot=off  SenseRDDot=off  SenseX=on  SenseY=on  SenseZ=on  SenseRad=off  SenseAzim=off  SenseDist=off  SenseInc=off  SenseXDot=off  SenseYDot=off  SenseZDot=off  SenseRadDot=off  SenseAzimDot=off  SenseDistDot=off  SenseIncDot=off  SenseXDDot=off  SenseYDDot=off  SenseZDDot=off  SenseRadDDot=off  SenseAzimDDot=off  SenseDistDDot=off  SenseIncDDot=off
  World1 : sm_lib/Frames and Transforms/World Frame
  Conn1 : PMIOPort  Side=Left
  R : Outport
  p : Outport  Port=2
  wires:
  Gain/1 -> p/1
  Selector/1 -> Gain/1
  Subsystem/2(R) -> Reshape/1
  Rotation Matrix to VRML Rotation1/1 -> R/1
  Reshape/1 -> Rotation Matrix to VRML Rotation1/1
  Subsystem/1(p) -> Selector/1
  connections:
  World1/RConn1 -- Transform Sensor/LConn1
  Transform Sensor/RConn1 -- Conn1/RConn1
  Transform Sensor/RConn4 -- Subsystem/LConn3
  Transform Sensor/RConn5 -- Subsystem/LConn4
  Transform Sensor/RConn2 -- Subsystem/LConn1
  Transform Sensor/RConn3 -- Subsystem/LConn2

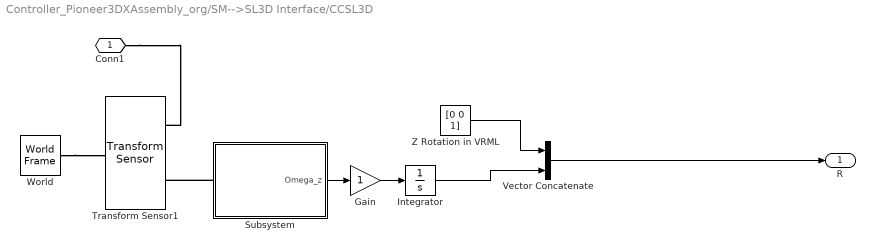
== system Controller_Pioneer3DXAssembly_org/SM-->SL3D Interface/CCSL3D ==
  Gain : Gain
  Integrator : Integrator
  Subsystem : Subsystem
  Transform Sensor1 : sm_lib/Frames and Transforms/Transform Sensor  MeasurementFrame=Base  SenseAngle=off  SenseAxis=off  SenseAngle1=off  SenseAngle2=off  SenseAngle3=off  SenseQ=off  SenseR=off  SenseOmegaX=off  SenseOmegaY=off  SenseOmegaZ=on  SenseOmega1=off  SenseOmega2=off  SenseOmega3=off  SenseQDot=off  SenseRDot=off  SenseAlphaX=off  SenseAlphaY=off  SenseAlphaZ=off  SenseAlpha1=off  SenseAlpha2=off  SenseAlpha3=off  SenseQDDot=off  SenseRDDot=off  SenseX=off  SenseY=off  SenseZ=off  SenseRad=off  SenseAzim=off  SenseDist=off  SenseInc=off  SenseXDot=off  SenseYDot=off  SenseZDot=off  SenseRadDot=off  SenseAzimDot=off  SenseDistDot=off  SenseIncDot=off  SenseXDDot=off  SenseYDDot=off  SenseZDDot=off  SenseRadDDot=off  SenseAzimDDot=off  SenseDistDDot=off  SenseIncDDot=off
  Vector Concatenate : Concatenate
  World : sm_lib/Frames and Transforms/World Frame
  Z Rotation in VRML : Constant  Value=[0 0 1]
  Conn1 : PMIOPort  Side=Left
  R : Outport
  wires:
  Vector Concatenate/1 -> R/1
  Z Rotation in VRML/1 -> Vector Concatenate/1
  Subsystem/1(Omega_z) -> Gain/1
  Integrator/1 -> Vector Concatenate/2
  Gain/1 -> Integrator/1
  connections:
  World/RConn1 -- Transform Sensor1/LConn1
  Subsystem/LConn1 -- Transform Sensor1/RConn2
  Conn1/RConn1 -- Transform Sensor1/RConn1

== system Controller_Pioneer3DXAssembly_org/SM-->SL3D Interface/CWSL3D ==
  Integrator : Integrator
  Subsystem : Subsystem
  Transform Sensor1 : sm_lib/Frames and Transforms/Transform Sensor  MeasurementFrame=Base  SenseAngle=off  SenseAxis=off  SenseAngle1=off  SenseAngle2=off  SenseAngle3=off  SenseQ=off  SenseR=off  SenseOmegaX=off  SenseOmegaY=off  SenseOmegaZ=on  SenseOmega1=off  SenseOmega2=off  SenseOmega3=off  SenseQDot=off  SenseRDot=off  SenseAlphaX=off  SenseAlphaY=off  SenseAlphaZ=off  SenseAlpha1=off  SenseAlpha2=off  SenseAlpha3=off  SenseQDDot=off  SenseRDDot=off  SenseX=off  SenseY=off  SenseZ=off  SenseRad=off  SenseAzim=off  SenseDist=off  SenseInc=off  SenseXDot=off  SenseYDot=off  SenseZDot=off  SenseRadDot=off  SenseAzimDot=off  SenseDistDot=off  SenseIncDot=off  SenseXDDot=off  SenseYDDot=off  SenseZDDot=off  SenseRadDDot=off  SenseAzimDDot=off  SenseDistDDot=off  SenseIncDDot=off
  Vector Concatenate : Concatenate
  Z Rotation in VRML : Constant  Value=[0 1 0]
  Conn1 : PMIOPort  Side=Left
  Conn2 : PMIOPort  Port=2  Side=Left
  R : Outport
  wires:
  Subsystem/1(Omega_z) -> Integrator/1
  Integrator/1 -> Vector Concatenate/2
  Z Rotation in VRML/1 -> Vector Concatenate/1
  Vector Concatenate/1 -> R/1
  connections:
  Conn2/RConn1 -- Transform Sensor1/LConn1
  Conn1/RConn1 -- Transform Sensor1/RConn1
  Subsystem/LConn1 -- Transform Sensor1/RConn2

== system Controller_Pioneer3DXAssembly_org/SM-->SL3D Interface/LWSL3D ==
  Integrator : Integrator
  Subsystem : Subsystem
  Transform Sensor1 : sm_lib/Frames and Transforms/Transform Sensor  MeasurementFrame=Base  SenseAngle=off  SenseAxis=off  SenseAngle1=off  SenseAngle2=off  SenseAngle3=off  SenseQ=off  SenseR=off  SenseOmegaX=off  SenseOmegaY=off  SenseOmegaZ=on  SenseOmega1=off  SenseOmega2=off  SenseOmega3=off  SenseQDot=off  SenseRDot=off  SenseAlphaX=off  SenseAlphaY=off  SenseAlphaZ=off  SenseAlpha1=off  SenseAlpha2=off  SenseAlpha3=off  SenseQDDot=off  SenseRDDot=off  SenseX=off  SenseY=off  SenseZ=off  SenseRad=off  SenseAzim=off  SenseDist=off  SenseInc=off  SenseXDot=off  SenseYDot=off  SenseZDot=off  SenseRadDot=off  SenseAzimDot=off  SenseDistDot=off  SenseIncDot=off  SenseXDDot=off  SenseYDDot=off  SenseZDDot=off  SenseRadDDot=off  SenseAzimDDot=off  SenseDistDDot=off  SenseIncDDot=off
  Vector Concatenate : Concatenate
  Y Rotation in VRML : Constant  Value=[0 1 0]
  Conn1 : PMIOPort  Side=Left
  Conn2 : PMIOPort  Port=2  Side=Left
  R : Outport
  wires:
  Vector Concatenate/1 -> R/1
  Y Rotation in VRML/1 -> Vector Concatenate/1
  Subsystem/1(Omega_z) -> Integrator/1
  Integrator/1 -> Vector Concatenate/2
  connections:
  Subsystem/LConn1 -- Transform Sensor1/RConn2
  Conn2/RConn1 -- Transform Sensor1/LConn1
  Conn1/RConn1 -- Transform Sensor1/RConn1

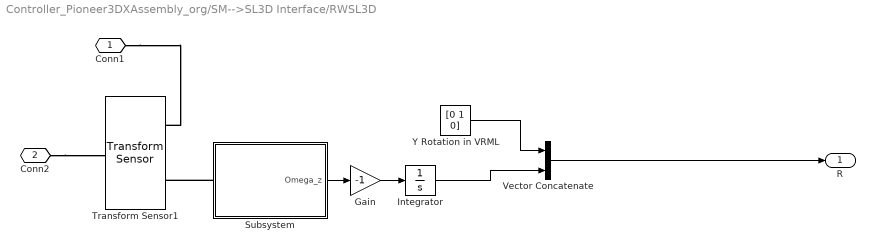
== system Controller_Pioneer3DXAssembly_org/SM-->SL3D Interface/RWSL3D ==
  Gain : Gain  Gain=-1
  Integrator : Integrator
  Subsystem : Subsystem
  Transform Sensor1 : sm_lib/Frames and Transforms/Transform Sensor  MeasurementFrame=Base  SenseAngle=off  SenseAxis=off  SenseAngle1=off  SenseAngle2=off  SenseAngle3=off  SenseQ=off  SenseR=off  SenseOmegaX=off  SenseOmegaY=off  SenseOmegaZ=on  SenseOmega1=off  SenseOmega2=off  SenseOmega3=off  SenseQDot=off  SenseRDot=off  SenseAlphaX=off  SenseAlphaY=off  SenseAlphaZ=off  SenseAlpha1=off  SenseAlpha2=off  SenseAlpha3=off  SenseQDDot=off  SenseRDDot=off  SenseX=off  SenseY=off  SenseZ=off  SenseRad=off  SenseAzim=off  SenseDist=off  SenseInc=off  SenseXDot=off  SenseYDot=off  SenseZDot=off  SenseRadDot=off  SenseAzimDot=off  SenseDistDot=off  SenseIncDot=off  SenseXDDot=off  SenseYDDot=off  SenseZDDot=off  SenseRadDDot=off  SenseAzimDDot=off  SenseDistDDot=off  SenseIncDDot=off
  Vector Concatenate : Concatenate
  Y Rotation in VRML : Constant  Value=[0 1 0]
  Conn1 : PMIOPort  Side=Left
  Conn2 : PMIOPort  Port=2  Side=Left
  R : Outport
  wires:
  Gain/1 -> Integrator/1
  Integrator/1 -> Vector Concatenate/2
  Subsystem/1(Omega_z) -> Gain/1
  Y Rotation in VRML/1 -> Vector Concatenate/1
  Vector Concatenate/1 -> R/1
  connections:
  Conn1/RConn1 -- Transform Sensor1/RConn1
  Conn2/RConn1 -- Transform Sensor1/LConn1
  Subsystem/LConn1 -- Transform Sensor1/RConn2

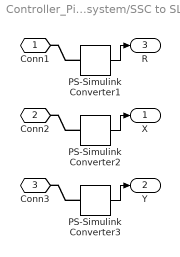
== system Controller_Pioneer3DXAssembly_org/Virtual Sensors Subsystem/SSC to SL ==
  PS-Simulink Converter1 : nesl_utility/PS-Simulink Converter  PhysicalDomain=network_engine_domain  SubClassName=ps_output  LeftPortType=input  RightPortType=output  PseudoPeriodic=off  Frequencies=[]  Unit=1  AffineConversion=off
  PS-Simulink Converter2 : nesl_utility/PS-Simulink Converter  PhysicalDomain=network_engine_domain  SubClassName=ps_output  LeftPortType=input  RightPortType=output  PseudoPeriodic=off  Frequencies=[]  Unit=1  AffineConversion=off
  PS-Simulink Converter3 : nesl_utility/PS-Simulink Converter  PhysicalDomain=network_engine_domain  SubClassName=ps_output  LeftPortType=input  RightPortType=output  PseudoPeriodic=off  Frequencies=[]  Unit=1  AffineConversion=off
  Conn1 : PMIOPort  Side=Left
  Conn2 : PMIOPort  Port=2  Side=Left
  Conn3 : PMIOPort  Port=3  Side=Left
  X : Outport
  Y : Outport  Port=2
  R : Outport  Port=3
  wires:
  PS-Simulink Converter3/1 -> Y/1
  PS-Simulink Converter1/1 -> R/1
  PS-Simulink Converter2/1 -> X/1
  connections:
  PS-Simulink Converter3/LConn1 -- Conn3/RConn1
  PS-Simulink Converter2/LConn1 -- Conn2/RConn1
  PS-Simulink Converter1/LConn1 -- Conn1/RConn1

== system Controller_Pioneer3DXAssembly_org/Virtual Sensors Subsystem/Virtual Sensors Lookup ==
  xR : Inport  OutDataTypeStr=double
  yR : Inport  Port=2  OutDataTypeStr=double
  2-D Lookup Table : Lookup_n-D  BreakpointsForDimension1=-1:0.001:1  BreakpointsForDimension2=-6:0.001:6  Table=World_LUT  RndMeth=Simplest  InputSameDT=on
  Sensors : Outport
  wires:
  2-D Lookup Table/1 -> Sensors/1
  xR/1 -> 2-D Lookup Table/1
  yR/1 -> 2-D Lookup Table/2

== system Controller_Pioneer3DXAssembly_org/Wheel Left/WheelMain_2_RIGID ==
  ReferenceFrame : sm_lib/Frames and Transforms/Reference Frame
  Solid : sm_lib/Body Elements/File Solid  ExtGeomFileName=WheelMain_Default_sldprt.STL  UnitType=FromFile  ExtGeomFileUnits=in  StepReaderType=HEX  ExportEntireGeometry=off  InertiaType=Custom  Mass=0.95054099999999997  MassUnits=kg  CenterOfMass=[6.6644881889763772 2.3641220472440942e-11 0.063999999999999987]  CenterOfMassUnits=in  MomentsOfInertia=[7.7667865335730646 4.0958211916423819 4.0958211916423819]  MomentsOfInertiaUnits=kg*in^2  ProductsOfInertia=[-2.8456041912083817e-11 2.5874201748403487e-11 1.023105896211792e-11]  ProductsOfInertiaUnits=kg*in^2  BasedOnType=Density  Density=1000  DensityUnits=kg/(m^3)  DoExposeReferenceFrame=on  SerializedFrames=<Frames/>  GraphicType=FromGeometry  MarkerShape=Sphere  MarkerSize=10  MarkerSizeUnits=m  GraphicVisPropType=SimpleVisualProperties  GraphicDiffuseColor=[0.792157 0.819608 0.933333]  GraphicSpecularColor=[0.5 0.5 0.5 1.0]  GraphicAmbientColor=[0.15 0.15 0.15 1.0]  GraphicEmissiveColor=[0.0 0.0 0.0 1.0]  GraphicShininess=75  GraphicOpacity=1
  Transform : sm_lib/Frames and Transforms/Rigid Transform  TranslationMethod=Cartesian  TranslationStandardOffset=0  TranslationLengthUnit=m  TranslationStandardAxis=+Z  TranslationCartesianOffset=[0.18929381000000001 -3.8310365150845058e-08 0.0016256173284423497]  TranslationROffset=0  TranslationROffsetUnits=m  TranslationZOffset=0  TranslationZOffsetUnits=m  TranslationThetaOffset=0  TranslationThetaOffsetUnits=deg  RotationMethod=ArbitraryAxis  RotationAngleUnits=rad  RotationStandardAxis=+Z  RotationAngle=2.0943951023931957  RotationArbitraryAxis=[-0.57735026918962562 -0.57735026918962584 0.57735026918962584]  FollAlignAxisA=+X  BaseAlignAxisA=+Y  FollAlignAxisB=+Y  BaseAlignAxisB=+Z  RotationSequenceAxes=FollowerAxes  RotationSequence=XYX  RotationSequenceAngles=[0 0 0]  RotationSequenceAnglesUnits=deg  RotationMatrix=[1 0 0; 0 1 0; 0 0 1]
  F : PMIOPort  Side=Left
  connections:
  Transform/RConn1 -- F/RConn1
  Transform/LConn1 -- ReferenceFrame/RConn1 -- Solid/RConn1
